simulink model "estTest_calibration"  (R2021b)
settings: Solver=FixedStepAuto  StartTime=0.0  StopTime=39.5  FixedStep=0.001  RelTol=1e-3
model workspace (MAT data in the model file):
  Ts = Simulink.Parameter
  Ts.Value = 0.001
  Ts.DataType = 'auto'
  Ts.Complexity = 'real'
  Ts.Dimensions = [1 1]
settings Model: Creator=kboxi  LastModifiedBy=boxingwang

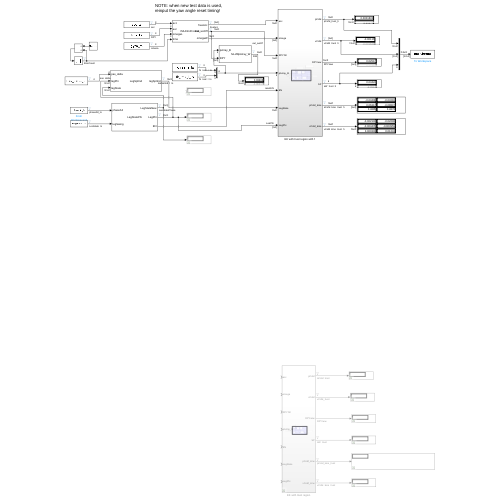
[thumbnail: Simulink's stored preview of the top-level diagram]
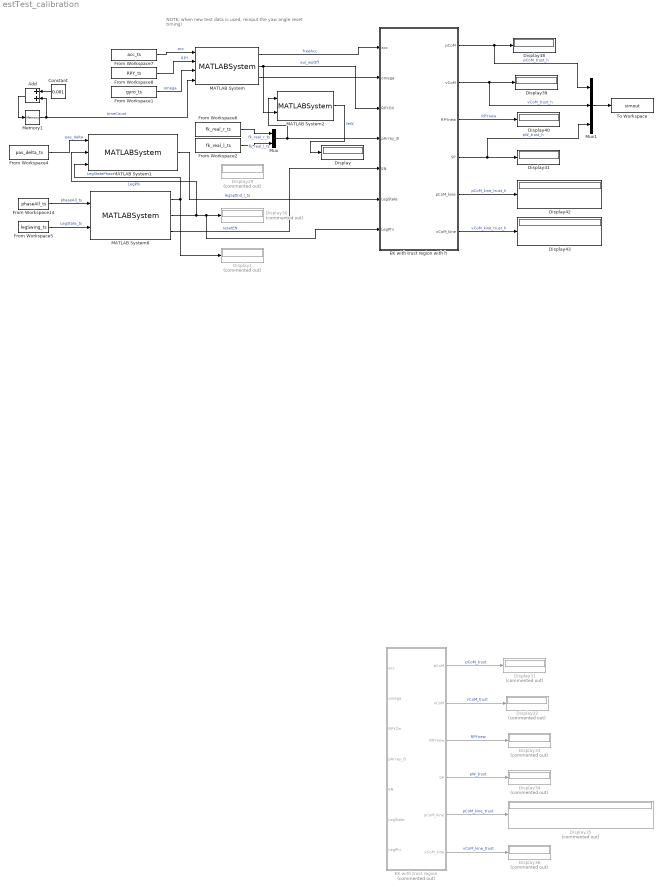
== system estTest_calibration ==
  note: NOTE: when new test data is used, reinput the yaw angle reset timing!
  Add : Sum
  Constant : Constant  Value=0.001
  Display{,38..43} (7 alike) : Display
  Display{1,29..36} (9 alike) : Display  Commented=on
  EK with trust region : Subsystem  Commented=on
  EK with trust region with h : Subsystem
  From Workspace1 : FromWorkspace  VariableName=gyro_ts  SampleTime=Ts
  From Workspace14 : FromWorkspace  VariableName=phaseAll_ts  SampleTime=Ts
  From Workspace2 : FromWorkspace  VariableName=fk_real_l_ts  SampleTime=Ts
  From Workspace4 : FromWorkspace  VariableName=pas_delta_ts  SampleTime=Ts
  From Workspace5 : FromWorkspace  VariableName=legSwing_ts  SampleTime=Ts
  From Workspace6 : FromWorkspace  VariableName=fk_real_r_ts  SampleTime=Ts
  From Workspace7 : FromWorkspace  VariableName=acc_ts  SampleTime=Ts
  From Workspace8 : FromWorkspace  VariableName=RPY_ts  SampleTime=Ts
  MATLAB System : MATLABSystem  System=IMUinfoProcess  offsetTriggerTime=5  SimulateUsing=Code generation
      mask Type: IMUinfoProcess
      mask Display:
      | disp('IMUinfoProcess');
      | port_label('input',1,'acc');
      | port_label('input',2,'eul');
      | port_label('input',3,'omegaL');
      | port_label('input',4,'time');
      | port_label('output',1,'freeAcc');
      | port_label('output',2,'Eul_woOff');
      | port_label('output',3,'omegaW');
  MATLAB System1 : MATLABSystem  System=LegSptInd  SimulateUsing=Code generation
      mask Type: LegSptInd
      mask Display:
      | disp('LegSptInd');
      | port_label('input',1,'pas_delta');
      | port_label('input',2,'legPhi');
      | port_label('input',3,'legState');
      | port_label('output',1,'legSptInd');
  MATLAB System2 : MATLABSystem  System=feL2W  SimulateUsing=Code generation
      mask Type: feL2W
      mask Display:
      | disp('feL2W');
      | port_label('input',1,'pArray_B');
      | port_label('input',2,'RPY');
      | port_label('output',1,'pArray_W');
  MATLAB System6 : MATLABSystem  System=LegStatePhi  maxPhiCount=500  SimulateUsing=Code generation
      mask Type: LegStatePhi
      mask Display:
      | disp('LegStatePhi');
      | port_label('input',1,'phaseAll');
      | port_label('input',2,'legSwing');
      | port_label('output',1,'LegStateNew');
      | port_label('output',2,'LegPhi');
      | port_label('output',3,'EN');
  Memory1 : Memory  InheritSampleTime=on
  Mux : Mux  Inputs=2
  Mux1 : Mux  Inputs=3
  To Workspace : ToWorkspace  VariableName=simout  SaveFormat=Structure With Time  SampleTime=-1
  wires:
  MATLAB System6/3 -> EK with trust region with h/5(EN)  "resetEN"
  From Workspace14/1 -> MATLAB System6/1  "phaseAll_ts"
  MATLAB System6/2 -> MATLAB System1/2, EK with trust region with h/7(LegPhi), Display30/1  "LegPhi"
  EK with trust region/1(pCoM) -> Display31/1  "pCoM_trust"
  EK with trust region/2(vCoM) -> Display32/1  "vCoM_trust"
  EK with trust region/3(RPYnew) -> Display33/1  "RPYnew"
  EK with trust region/4(SP) -> Display34/1  "pW_trust"
  EK with trust region/5(pCoM_kine) -> Display35/1  "pCoM_kine_trust"
  EK with trust region/6(vCoM_kine) -> Display36/1  "vCoM_kine_trust"
  EK with trust region with h/1(pCoM) -> Mux1/1, Display38/1  "pCoM_trust_h"
  EK with trust region with h/2(vCoM) -> Mux1/2, Display39/1  "vCoM_trust_h"
  EK with trust region with h/3(RPYnew) -> Display40/1  "RPYnew"
  EK with trust region with h/4(SP) -> Mux1/3, Display41/1  "pW_trust_h"
  EK with trust region with h/5(pCoM_kine) -> Display42/1  "pCoM_kine_trust_h"
  EK with trust region with h/6(vCoM_kine) -> Display43/1  "vCoM_kine_trust_h"
  From Workspace5/1 -> MATLAB System6/2  "LegState_ts"
  From Workspace7/1 -> MATLAB System/1  "acc"
  From Workspace8/1 -> MATLAB System/2  "RPY"
  MATLAB System/1 -> EK with trust region with h/1(acc)  "freeAcc"
  From Workspace6/1 -> Mux/1  "fk_real_r_ts"
  From Workspace2/1 -> Mux/2  "fk_real_l_ts"
  Mux/1 -> MATLAB System2/1, EK with trust region with h/4(pArray_B)
  Memory1/1 -> MATLAB System/4, Add/2  "timeCount"
  Add/1 -> Memory1/1
  Constant/1 -> Add/1
  MATLAB System/2 -> EK with trust region with h/3(RPYOri), MATLAB System2/2  "eul_woOff"
  From Workspace1/1 -> MATLAB System/3  "omega"
  MATLAB System/3 -> EK with trust region with h/2(omega)
  Mux1/1 -> To Workspace/1
  MATLAB System1/1 -> EK with trust region with h/6(LegState)  "legSptInd_l_ts"
  MATLAB System6/1 -> Display1/1, MATLAB System1/3  "LegStatePhase"
  From Workspace4/1 -> MATLAB System1/1  "pas_delta"
  MATLAB System2/1 -> Display/1  "feW"

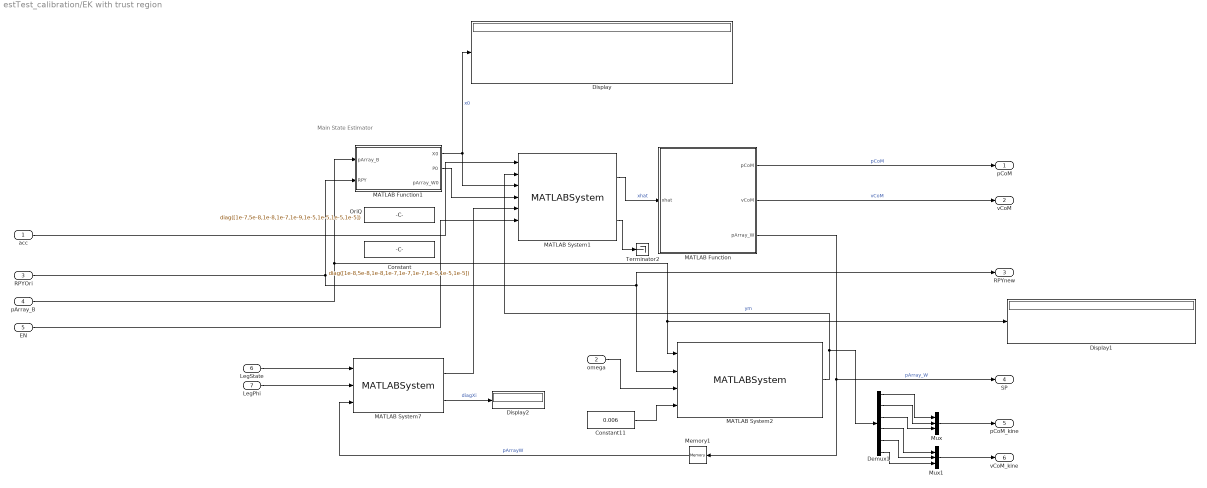
== system estTest_calibration/EK with trust region ==
  note: Main State Estimator
  acc : Inport
  omega : Inport  Port=2
  RPYOri : Inport  Port=3
  pArray_B : Inport  Port=4
  EN : Inport  Port=5
  LegState : Inport  Port=6
  LegPhi : Inport  Port=7
  Constant : Constant  Value=diag([1e-8,5e-8,1e-8,1e-7,1e-7,1e-7,1e-5,1e-5,1e-5])
  Constant11 : Constant  Value=0.006
  Demux1 : Demux  Outputs=6
  Display : Display
  Display1 : Display
  Display2 : Display
  MATLAB Function : MATLAB Function  TreatAsAtomicUnit=on
  MATLAB Function1 : MATLAB Function  TreatAsAtomicUnit=on
  MATLAB System1 : MATLABSystem  System=KalmanFilter_DIY_TrustRegion_h  dt=0.006  Q_wPCoM=[ 1e-7; 5e-8; 1e-8 ]  Q_wVCoM=[ 1e-7, 1e-9, 1e-5 ]  Q_wfeW=ones( 12, 1 ) * (1e-6)  Q_waL=ones( 3, 1 ) * (1e-3)  R_wfeL=ones( 12, 1 ) * (1e-6)  R_wdfeL=ones( 12, 1 ) * (1e-3)  R_wh=ones( 4, 1 ) * (1e-6)  SimulateUsing=Code generation
      mask Type: KalmanFilter_DIY_TrustRegion_h
      mask Display:
      | disp('KalmanFilter_DIY_TrustRegion_h');
      | port_label('input',1,'u');
      | port_label('input',2,'y');
      | port_label('input',3,'x0');
      | port_label('input',4,'p0');
      | port_label('input',5,'Xi');
      | port_label('input',6,'Xih');
      | port_label('input',7,'Reset');
      | port_label('output',1,'xhat');
      | port_label('output',2,'P');
  MATLAB System2 : MATLABSystem  System=estY_byKine  SimulateUsing=Code generation
      mask Type: estY_byKine
      mask Display:
      | disp('estY_byKine');
      | port_label('input',1,'pArray_B');
      | port_label('input',2,'RPY');
      | port_label('input',3,'OmegaW');
      | port_label('input',4,'dt');
      | port_label('output',1,'ym');
  MATLAB System7 : MATLABSystem  System=TrustRegion  k=10  Cphi_W=0.1  Cz_kp=50000  Cz_kn=50000  SimulateUsing=Code generation
      mask Type: TrustRegion
      mask Display:
      | disp('TrustRegion');
      | port_label('input',1,'LegState');
      | port_label('input',2,'LegPhi');
      | port_label('input',3,'pW');
      | port_label('output',1,'Xi');
      | port_label('output',2,'diagXi');
  Memory1 : Memory  InitialCondition=zeros(12,1)  InheritSampleTime=on
  Mux : Mux  Inputs=3
  Mux1 : Mux  Inputs=3
  OriQ : Constant  Value=diag([1e-7,5e-8,1e-8,1e-7,1e-9,1e-5,1e-5,1e-5,1e-5])
  Terminator2 : Terminator
  pCoM : Outport
  vCoM : Outport  Port=2
  RPYnew : Outport  Port=3
  SP : Outport  Port=4
  pCoM_kine : Outport  Port=5
  vCoM_kine : Outport  Port=6
  wires:
  MATLAB System2/1 -> MATLAB System1/2, Demux1/1  "ym"
  MATLAB System1/1 -> MATLAB Function/1(xhat)  "xhat"
  pArray_B/1 -> MATLAB Function1/1(pArray_B), Display1/1, MATLAB System2/1
  MATLAB Function1/1(X0) -> MATLAB System1/3, Display/1  "x0"
  MATLAB Function/1(pCoM) -> pCoM/1  "pCoM"
  MATLAB Function/2(vCoM) -> vCoM/1  "vCoM"
  MATLAB Function1/2(P0) -> MATLAB System1/4
  MATLAB Function/3(pArray_W) -> SP/1, Memory1/1  "pArray_W"
  acc/1 -> MATLAB System1/1
  Demux1/1 -> Mux/1
  Demux1/2 -> Mux/2
  Demux1/3 -> Mux/3
  Demux1/4 -> Mux1/1
  Demux1/5 -> Mux1/2
  Demux1/6 -> Mux1/3
  Mux/1 -> pCoM_kine/1
  Mux1/1 -> vCoM_kine/1
  MATLAB System1/2 -> Terminator2/1
  RPYOri/1 -> MATLAB Function1/2(RPY), RPYnew/1, MATLAB System2/2
  LegState/1 -> MATLAB System7/1
  LegPhi/1 -> MATLAB System7/2
  Memory1/1 -> MATLAB System7/3  "pArrayW"
  MATLAB System7/1 -> MATLAB System1/5
  EN/1 -> MATLAB System1/6
  MATLAB System7/2 -> Display2/1  "diagXi"
  Constant11/1 -> MATLAB System2/4
  omega/1 -> MATLAB System2/3

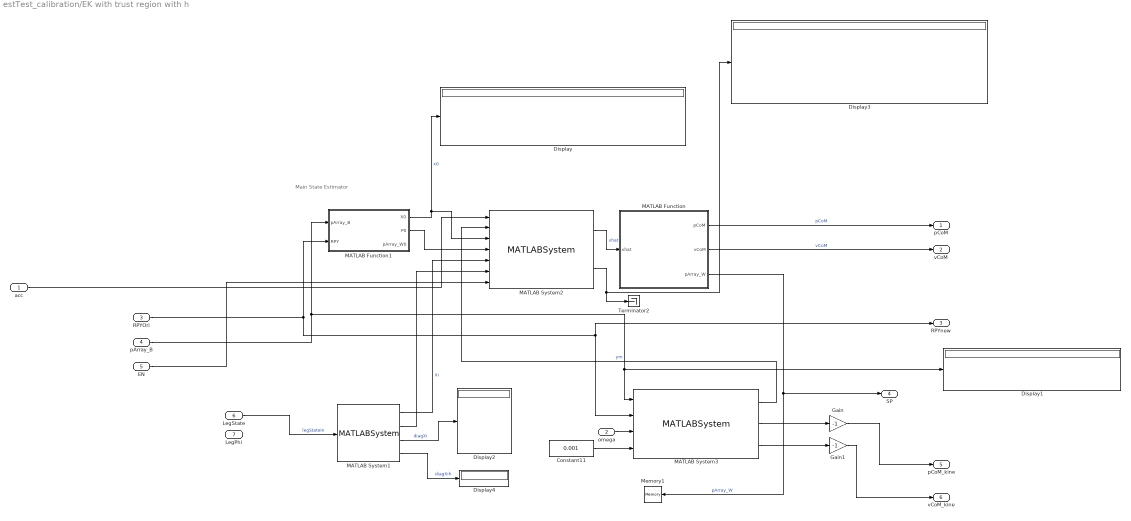
== system estTest_calibration/EK with trust region with h ==
  note: Main State Estimator
  acc : Inport
  omega : Inport  Port=2
  RPYOri : Inport  Port=3
  pArray_B : Inport  Port=4
  EN : Inport  Port=5
  LegState : Inport  Port=6
  LegPhi : Inport  Port=7
  Constant11 : Constant  Value=0.001
  Display{,1..4} (5 alike) : Display
  Gain : Gain  Gain=-1
  Gain1 : Gain  Gain=-1
  MATLAB Function : MATLAB Function  TreatAsAtomicUnit=on
  MATLAB Function1 : MATLAB Function  TreatAsAtomicUnit=on
  MATLAB System1 : MATLABSystem  System=TrustRegion_h_v2  k_few=100  k_fez2zero=100  SimulateUsing=Code generation
      mask Type: TrustRegion_h_v2
      mask Display:
      | disp('TrustRegion_h_v2');
      | port_label('input',1,'LegState');
      | port_label('output',1,'Xi');
      | port_label('output',2,'Xih');
      | port_label('output',3,'diagXi');
      | port_label('output',4,'diagXih');
  MATLAB System2 : MATLABSystem  System=KalmanFilter_DIY_TrustRegion_h  dt=0.001  Q_wPCoM=[ 1e-2; 1e-2; 1 ]*(1e-7)  Q_wVCoM=[ 1, 1, 1 ]*(1e-7)  Q_wfeW=ones(6, 1 ) * (1e-6)  Q_waL=[1.5298;1.5967;2.5534] * (1e-10)  Q_wau=[ 2, 2, 5 ] * (1e-4)  R_wfeL=[1.46,1.3e-5,8.7e-1,2.5,3.7e-5,3.2e-5] * (1e-9)  R_wdfeL=ones( 6, 1 ) * (1e-3)  R_wh=ones( 2, 1 ) * (1e-6)  SimulateUsing=Code generation
      mask Type: KalmanFilter_DIY_TrustRegion_h
      mask Display:
      | disp('KalmanFilter_DIY_TrustRegion_h');
      | port_label('input',1,'u');
      | port_label('input',2,'y');
      | port_label('input',3,'x0');
      | port_label('input',4,'p0');
      | port_label('input',5,'Xi');
      | port_label('input',6,'Xih');
      | port_label('input',7,'Reset');
      | port_label('output',1,'xhat');
      | port_label('output',2,'P');
  MATLAB System3 : MATLABSystem  System=estY_byKine_h  SimulateUsing=Code generation
      mask Type: estY_byKine_h
      mask Display:
      | disp('estY_byKine_h');
      | port_label('input',1,'pArray_B');
      | port_label('input',2,'RPY');
      | port_label('input',3,'OmegaW');
      | port_label('input',4,'dt');
      | port_label('output',1,'ym');
      | port_label('output',2,'pArray_W_kine');
      | port_label('output',3,'vArray_W_kine');
  Memory1 : Memory  InitialCondition=zeros(6,1)  InheritSampleTime=on
  Terminator2 : Terminator
  pCoM : Outport
  vCoM : Outport  Port=2
  RPYnew : Outport  Port=3
  SP : Outport  Port=4
  pCoM_kine : Outport  Port=5
  vCoM_kine : Outport  Port=6
  wires:
  omega/1 -> MATLAB System3/3
  Constant11/1 -> MATLAB System3/4
  MATLAB System1/3 -> Display2/1  "diagXi"
  EN/1 -> MATLAB System2/7
  MATLAB System1/1 -> MATLAB System2/5  "Xi"
  LegState/1 -> MATLAB System1/1  "legStateIn"
  RPYOri/1 -> MATLAB System3/2, RPYnew/1, MATLAB Function1/2(RPY)
  MATLAB System2/2 -> Display3/1, Terminator2/1
  acc/1 -> MATLAB System2/1
  MATLAB Function/3(pArray_W) -> Memory1/1, SP/1  "pArray_W"
  MATLAB Function1/2(P0) -> MATLAB System2/4
  MATLAB Function/2(vCoM) -> vCoM/1  "vCoM"
  MATLAB Function/1(pCoM) -> pCoM/1  "pCoM"
  MATLAB Function1/1(X0) -> MATLAB System2/3, Display/1  "x0"
  pArray_B/1 -> MATLAB System3/1, Display1/1, MATLAB Function1/1(pArray_B)
  MATLAB System2/1 -> MATLAB Function/1(xhat)  "xhat"
  MATLAB System3/1 -> MATLAB System2/2  "ym"
  MATLAB System1/2 -> MATLAB System2/6
  MATLAB System3/2 -> Gain/1
  MATLAB System3/3 -> Gain1/1
  Gain/1 -> pCoM_kine/1
  Gain1/1 -> vCoM_kine/1
  MATLAB System1/4 -> Display4/1  "diagXih"

== matlab function estTest_calibration/EK with trust region/MATLAB Function ==
  data: xhat input size=[21,1]; pCoM output size=[3,1]; vCoM output size=[3,1]; pArray_W output
function [pCoM,vCoM,pArray_W] = fcn(xhat)
% pB the CoM position in the world coordinate
% vB the CoM velocity
% Wpi the foot-end position in the world coordinate
pCoM=[xhat(1);xhat(2);xhat(3)];
vCoM=[xhat(4);xhat(5);xhat(6)];
pArray_W=reshape(xhat(7:18),12,1);

== matlab function estTest_calibration/EK with trust region/MATLAB Function1 ==
  data: pArray_B input; RPY input; X0 output; P0 output; pArray_W0 output
function [X0,P0,pArray_W0]=fcn(pArray_B,RPY)
% NOTE: pArray_W0 is calculated without the value of yaw angle!!!
Ry=[cos(RPY(2)),0,sin(RPY(2));
    0,1,0;
    -sin(RPY(2)),0,cos(RPY(2))];
Rx=[1,0,0;
    0,cos(RPY(1)),-sin(RPY(1));
    0,sin(RPY(1)),cos(RPY(1))];
pArray_B=reshape(pArray_B,3,4)/1000;
pArray_float=Ry*Rx*pArray_B; % foot-end position in floating coordinate
zOff=-min(pArray_float(3,:));
temp=pArray_float+[0;0;zOff]*[1,1,1,1];
pCoM=[0;0;zOff];
vCoM=[0;0;0];
abar=[0;0;0];
pArray_W0=[temp(:,1);temp(:,2);temp(:,3);temp(:,4)];
X0=[pCoM;vCoM;pArray_W0;abar];
P0=eye(21)*10^-3;

== matlab function estTest_calibration/EK with trust region with h/MATLAB Function ==
  data: xhat input size=[15,1]; pCoM output size=[3,1]; vCoM output size=[3,1]; pArray_W output
function [pCoM,vCoM,pArray_W] = fcn(xhat)
% pB the CoM position in the world coordinate
% vB the CoM velocity
% Wpi the foot-end position in the world coordinate
pCoM=[xhat(1);xhat(2);xhat(3)];
vCoM=[xhat(4);xhat(5);xhat(6)];
pArray_W=reshape(xhat(7:12),6,1);

== matlab function estTest_calibration/EK with trust region with h/MATLAB Function1 ==
  data: pArray_B input; RPY input; X0 output size=[15,1]; P0 output size=[15,15]; pArray_W0 output
function [X0,P0,pArray_W0]=fcn(pArray_B,RPY)
% NOTE: pArray_W0 is calculated without the value of yaw angle!!!
Ry=[cos(RPY(2)),0,sin(RPY(2));
    0,1,0;
    -sin(RPY(2)),0,cos(RPY(2))];
Rx=[1,0,0;
    0,cos(RPY(1)),-sin(RPY(1));
    0,sin(RPY(1)),cos(RPY(1))];
pArray_B=reshape(pArray_B,3,2);
pArray_float=Ry*Rx*pArray_B; % foot-end position in floating coordinate
zOff=-sum(pArray_float(3,:))/2;
temp=pArray_float+[0;0;zOff]*[1,1];
pCoM=[0;0;zOff];
vCoM=[0;0;0];
abar=[0;0;0];
pArray_W0=[temp(:,1);temp(:,2)];
X0=[pCoM;vCoM;pArray_W0;abar];
P0=eye(length(X0))*10^-3;
